simulink model "FOUR_STEP_BDS"  (R2019b)
settings: Solver=VariableStepAuto  StartTime=0.0  StopTime=10.0  RelTol=1e-3
undefined symbols (not defined in the file): timeStep
settings Model: Creator=simone  LastModifiedBy=simone

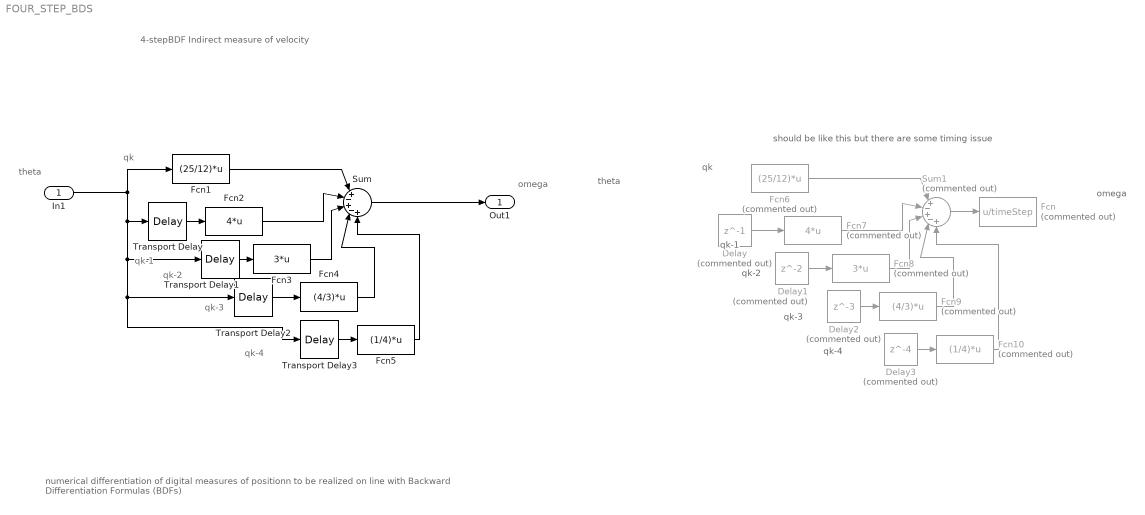
== system FOUR_STEP_BDS ==
  note: should be like this but there are some timing issue
  note: omega
  note: theta
  note: qk-4
  note: qk-3
  note: qk-2
  note: qk-1
  note: qk
  note: 4-stepBDF
      | Indirect measure of velocity
  note: numerical differentiation of digital measures of positionn to be realized on line with Backward Differentiation Formulas (BDFs)
  note: qk-1
  note: qk-3
  note: qk-2
  note: qk
  note: qk-4
  note: theta
  note: omega
  In1 : Inport
  Delay : Delay  Commented=on  DelayLength=1  InitialCondition=0  SampleTime=timeStep
  Delay1 : Delay  Commented=on  InitialCondition=0  SampleTime=timeStep
  Delay2 : Delay  Commented=on  DelayLength=3  InitialCondition=0  SampleTime=timeStep
  Delay3 : Delay  Commented=on  DelayLength=4  InitialCondition=0  SampleTime=timeStep
  Fcn : Fcn  Commented=on  Expr=u/timeStep
  Fcn1 : Fcn  Expr=(25/12)*u
  Fcn10 : Fcn  Commented=on  Expr=(1/4)*u
  Fcn2 : Fcn  Expr=4*u
  Fcn3 : Fcn  Expr=3*u
  Fcn4 : Fcn  Expr=(4/3)*u
  Fcn5 : Fcn  Expr=(1/4)*u
  Fcn6 : Fcn  Commented=on  Expr=(25/12)*u
  Fcn7 : Fcn  Commented=on  Expr=4*u
  Fcn8 : Fcn  Commented=on  Expr=3*u
  Fcn9 : Fcn  Commented=on  Expr=(4/3)*u
  Sum : Sum  Inputs=|+-+-+
  Sum1 : Sum  Commented=on  Inputs=|+-+-+
  Transport Delay : TransportDelay
  Transport Delay1 : TransportDelay  DelayTime=2
  Transport Delay2 : TransportDelay  DelayTime=3
  Transport Delay3 : TransportDelay  DelayTime=4
  Out1 : Outport
  wires:
  In1/1 -> Transport Delay/1, Transport Delay1/1, Transport Delay3/1, Transport Delay2/1, Fcn1/1
  Fcn1/1 -> Sum/1
  Fcn2/1 -> Sum/2
  Fcn3/1 -> Sum/3
  Fcn4/1 -> Sum/4
  Fcn5/1 -> Sum/5
  Transport Delay/1 -> Fcn2/1
  Transport Delay1/1 -> Fcn3/1
  Transport Delay2/1 -> Fcn4/1
  Transport Delay3/1 -> Fcn5/1
  Delay/1 -> Fcn7/1
  Delay2/1 -> Fcn9/1
  Delay1/1 -> Fcn8/1
  Delay3/1 -> Fcn10/1
  Fcn9/1 -> Sum1/4
  Fcn6/1 -> Sum1/1
  Fcn8/1 -> Sum1/3
  Fcn7/1 -> Sum1/2
  Sum1/1 -> Fcn/1
  Fcn10/1 -> Sum1/5
  Sum/1 -> Out1/1
